simulink model "motor_real"  (R2017a)
settings: Solver=VariableStepAuto  StartTime=0.0  StopTime=5  MaxStep=1e-4  RelTol=1e-3
libraries: powerlib x5, powerlib_meascontrol x1
settings Model: Creator=Administrator  LastModifiedBy=Administrator

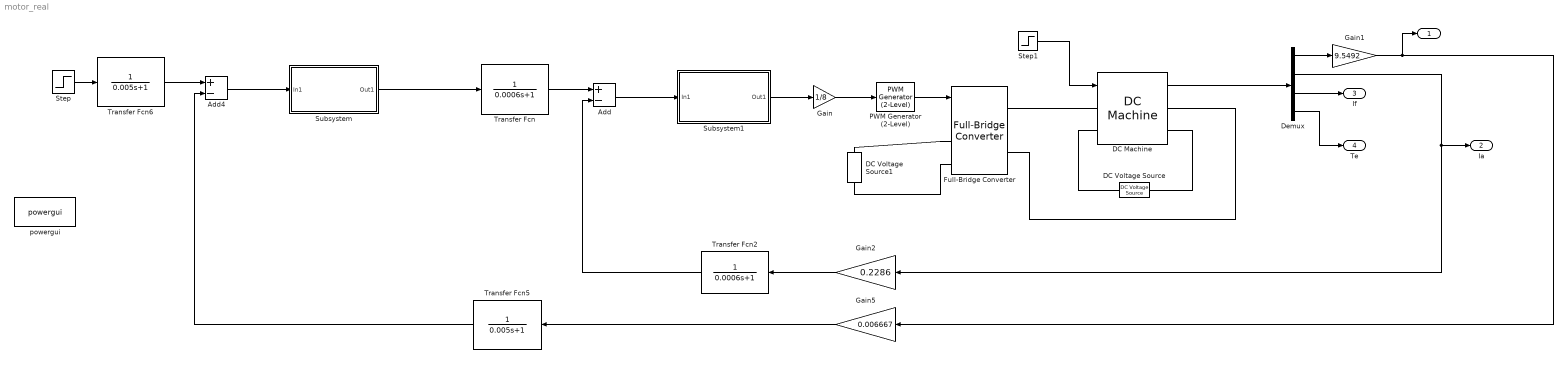
== system motor_real ==
  Add : Sum  Inputs=+-
  Add4 : Sum  Inputs=+-
  DC Machine : powerlib/Machines/DC Machine  PresetModel=No  MechanicalLoad=Torque TL  FieldType=Wound  ShowDetailedParameters=on  MeasurementBus=off  RLa="[ 1.2  0.016]"  RLf="[ 183.3333  91]"  Laf=1.0557  MachineConstant=Torque constant (N.m/A)  Ke=1.8  Kt=1.8  J=0.0102  Bm=0  Tf=0  w0=0  Ifinit=1.2  TsPowergui=0  TsBlock=-1
  DC Voltage Source : powerlib/Electrical Sources/DC Voltage Source  Amplitude=220  Measurements=None
  DC Voltage Source1 : powerlib/Electrical Sources/DC Voltage Source  Amplitude=220  Measurements=None
  Demux : Demux
  Full-Bridge Converter : powerlib/Power Electronics/Full-Bridge Converter  ModelType=Switching devices  Ron=1e-3  Rs=1e6  Cs=inf  Vforward=[0,0]  Ron_Diode=1e-3  Rs_Diode=1e6  Cs_Diode=inf  Vf_Diode=1e-3  Rs_CurrentSource=inf
      settings: SourceProductName=Simscape Power Systems  SourceProductBaseCode=PS
  Gain : Gain  Gain=1/8
  Gain1 : Gain  Gain=9.5492
  Gain2 : Gain  Gain=0.2286
  Gain5 : Gain  Gain=0.006667
  PWM Generator (2-Level) : powerlib_meascontrol/Pulse & Signal Generators/PWM Generator (2-Level)  ModulatorType=Single-phase full-bridge - Bipolar modulation (4 pulses)  ModulatorMode=Unsynchronized  Fc=1000  Pc=0  nF=27  MinMax="[ -1  1 ]"  SamplingTechnique=Natural  ModulatingSignals=off  m=0.8  Freq=60  Phase=0  Ts=0  ShowCarrierOutport=off
      settings: SourceProductName=Simscape Power Systems
  Step : Step  Time=0  After=10  SampleTime=0
  Step1 : Step  Time=2.5  Before=0.02395  After=22.2  SampleTime=0
  Subsystem : Subsystem
  Subsystem1 : Subsystem
  Transfer Fcn : TransferFcn  Denominator=[0.0006 1]
  Transfer Fcn2 : TransferFcn  Denominator=[0.0006 1]
  Transfer Fcn5 : TransferFcn  Denominator=[0.005 1]
  Transfer Fcn6 : TransferFcn  Denominator=[0.005 1]
  powergui : powerlib/powergui  Priority=1  SimulationMode=Continuous  SampleTime=50e-6  frequency=60  Iterations=50  frequencyindice=0  Pbase=100e6  ErrMax=1e-4  UnitsV=kV  UnitsW=MW  buscounter=0  FunctionMessages=off  echomessages=off  EnableUseOfTLC=off  CurrentSourceSwitches=off  DisableSnubberDevices=off  DisableRonSwitches=off  DisableVfSwitches=off  DisplayEquations=off  SolverType=Tustin/Backward Euler (TBE)  Interpol=off  ExternalGateDelay=off  methode=off  Ts=100  x0status=blocks  SPID=on  SwTol=0  HookPort=off  RestoreLinks=warning  ResistiveCurrentMeasurement=off  Frange=[0:2:500]  Ylog=off  Xlog=on  ShowGrid=off  save=off  variable=ZData  structure=0  ZoomFFT=off  StartTime=0.0  cycles=1  DisplayStyle=1  fundamental=60  FreqAxis=off  MaxFrequency=1000  frequencyindicesteady=1  RmsSteady=1  display=off
  " " : Outport  SignalName=n
  Ia : Outport  Port=2
  If : Outport  Port=3
  Te : Outport  Port=4
  wires:
  Transfer Fcn5/1 -> Add4/2
  Transfer Fcn6/1 -> Add4/1
  Gain2/1 -> Transfer Fcn2/1
  Transfer Fcn/1 -> Add/1
  Gain5/1 -> Transfer Fcn5/1
  Step/1 -> Transfer Fcn6/1
  Transfer Fcn2/1 -> Add/2
  Add4/1 -> Subsystem/1(In1)
  Subsystem/1(Out1) -> Transfer Fcn/1
  Add/1 -> Subsystem1/1(In1)
  Gain/1 -> PWM Generator (2-Level)/1
  Subsystem1/1(Out1) -> Gain/1
  PWM Generator (2-Level)/1 -> Full-Bridge Converter/1
  DC Machine/1 -> Demux/1
  Step1/1 -> DC Machine/1
  Demux/4 -> Te/1
  Demux/1 -> Gain1/1
  Demux/2 -> Ia/1, Gain2/1
  Demux/3 -> If/1
  Gain1/1 -> " "/1, Gain5/1
  connections:
  Full-Bridge Converter/RConn1 -- DC Machine/LConn1
  Full-Bridge Converter/RConn2 -- DC Machine/RConn1
  DC Voltage Source/RConn1 -- DC Machine/LConn2
  DC Machine/RConn2 -- DC Voltage Source/LConn1
  Full-Bridge Converter/LConn1 -- DC Voltage Source1/RConn1
  DC Voltage Source1/LConn1 -- Full-Bridge Converter/LConn2

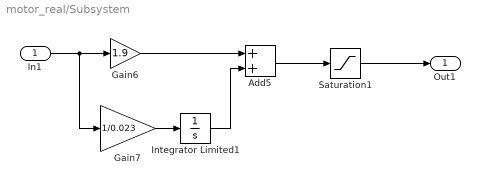
== system motor_real/Subsystem ==
  In1 : Inport
  Add5 : Sum
  Gain6 : Gain  Gain=1.9
  Gain7 : Gain  Gain=1/0.023
  Integrator Limited1 : Integrator  LimitOutput=on  UpperSaturationLimit=15  LowerSaturationLimit=-15
  Saturation1 : Saturate  UpperLimit=8  LowerLimit=-8
  Out1 : Outport
  wires:
  Integrator Limited1/1 -> Add5/2
  Gain7/1 -> Integrator Limited1/1
  Gain6/1 -> Add5/1
  Add5/1 -> Saturation1/1
  Saturation1/1 -> Out1/1
  In1/1 -> Gain7/1, Gain6/1

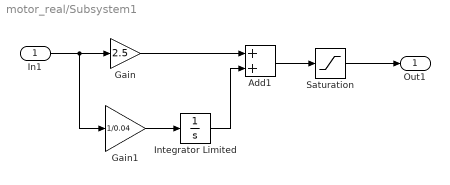
== system motor_real/Subsystem1 ==
  In1 : Inport
  Add1 : Sum
  Gain : Gain  Gain=2.5
  Gain1 : Gain  Gain=1/0.04
  Integrator Limited : Integrator  LimitOutput=on  UpperSaturationLimit=15  LowerSaturationLimit=-15
  Saturation : Saturate  UpperLimit=8  LowerLimit=-8
  Out1 : Outport
  wires:
  Add1/1 -> Saturation/1
  Gain1/1 -> Integrator Limited/1
  Gain/1 -> Add1/1
  Integrator Limited/1 -> Add1/2
  In1/1 -> Gain1/1, Gain/1
  Saturation/1 -> Out1/1
